simulink model "AcO_Ctrl_Geometric_headless_R2016a"  (R2016a)
settings: Solver=FixedStepDiscrete  StartTime=0.0  StopTime=simulation_duration  FixedStep=Ts  RelTol=1e-3
values from neighbouring files (symbols this model uses):
  M1_BeMo_d = zeros(7,M1_n_mode)    [AcO_Ctrl_headless_cfg.m]    (also in agws_cfg.m = 1e-6*bsxfun(@times,randn(7,M1_n_mode),scale); agws_fastTT_cfg.m = 1e-6*bsxfun(@times,randn(7,M1_n_mode),scale))
  M1_RiBo_d = zeros(7,6)    [AcO_Ctrl_headless_cfg.m]    (also in agws_cfg.m = [M1_Txyz0 M1_Rxyz0]; agws_fastTT_cfg.m = [M1_Txyz0 M1_Rxyz0])
  M2_RiBo_d = zeros(7,6)    [AcO_Ctrl_headless_cfg.m]    (also in agws_cfg.m = [M2_Txyz0 M2_Rxyz0]; agws_fastTT_cfg.m = [M2_Txyz0 M2_Rxyz0])
  Ts = 1/fs    (= 0.002)    [AcO_Ctrl_headless_cfg.m]    (also in agws_fastTT_cfg.m = 0.005)
undefined symbols (not defined in the file or in its folder): Az_C, CG2Hp, CG2Hp_S7, El_C, Fsmm, GIR_C, Hp2CG_f, Hp2CG_f_S7, HPdtf, HpK, KM2, M2_actdyn, M2_CG2Hp, M_LOS, MIMO_C, PTT2act, PTT2act_even, Q, sysd, TT2act, TT2act_even
undefined symbols (not defined in the file): on_axis_src_outputs
libraries: CEO x2
(part 2 of 6)

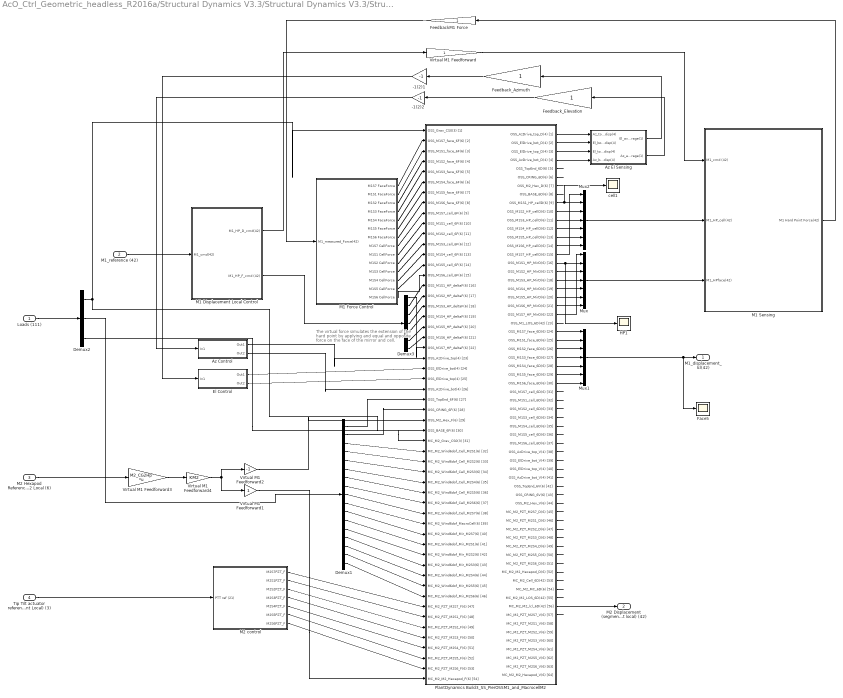
== system AcO_Ctrl_Geometric_headless_R2016a/Structural Dynamics V3.3/Structural Dynamics V3.3/Structural Dynamics Plus CL Az El M1 force ==
  note: The virtual force simulates the extension
      | of the hard point by applying and equal and
      | opposite force on the face of the mirror and cell.
  Loads (111) : Inport
  M1_reference (42) : Inport  Port=2
  M2 Hexapod Reference M2 Local (6) : Inport  Port=3
  Tip Tilt actuator reference (segment Local) (3) : Inport  Port=4
  -1(2)1 : Gain  Gain=-1
  -1(2)2 : Gain  Gain=-1
  Az Control : Subsystem
  Az El Sensing : Subsystem
  Demux1 : Demux  Outputs=6*ones(17,1)
  Demux2 : Demux  Outputs=[3,102,6]
  Demux3 : Demux  Outputs=6*ones(7,1)
  El Control : Subsystem
  Face5 : Scope
  FeedbackM1 Force : Gain
  Feedback_Azimuth : Gain
  Feedback_Elevation : Gain
  HP1 : Scope
  M1 Displacement Local Control : Subsystem
  M1 Force Control : Subsystem
  M1 Sensing : Subsystem
  M2 control : Subsystem
  Mux : Mux  Inputs=6*ones(7,1)
  Mux1 : Mux  Inputs=6*ones(7,1)
  Mux2 : Mux  Inputs=6*ones(7,1)
  PlantDynamics Build3_SS_PierOSSM1_and_MacrocellM2 : Subsystem
  Virtual M1 Feedforward : Gain
  Virtual M1 Feedforward1 : Gain
  Virtual M1 Feedforward2 : Gain  Gain=-1
  Virtual M1 Feedforward3 : Gain  Gain=M2_CG2Hp  Multiplication=Matrix(K*u)
  Virtual M1 Feedforward4 : Gain  Gain=KM2
  cell1 : Scope
  M1_displacement_lcl(42) : Outport
  M2 Displacement (segment local) (42) : Outport  Port=2
  wires:
  Loads (111)/1 -> Demux2/1
  M2 Hexapod Reference M2 Local (6)/1 -> Virtual M1 Feedforward3/1
  PlantDynamics Build3_SS_PierOSSM1_and_MacrocellM2/38(OSS_AzDrive_top_V(4) [38]) -> ?
  Virtual M1 Feedforward4/1 -> Virtual M1 Feedforward1/1, Virtual M1 Feedforward2/1
  Demux1/1 -> PlantDynamics Build3_SS_PierOSSM1_and_MacrocellM2/27(OSS_TopEnd_6F(6) [27])
  M2 control/7(M2S6PZT_F) -> PlantDynamics Build3_SS_PierOSSM1_and_MacrocellM2/53(MC_M2_PZT_M2S6_F(6) [53])
  M2 control/6(M2S5PZT_F) -> PlantDynamics Build3_SS_PierOSSM1_and_MacrocellM2/52(MC_M2_PZT_M2S5_F(6) [52])
  M2 control/5(M2S4PZT_F) -> PlantDynamics Build3_SS_PierOSSM1_and_MacrocellM2/51(MC_M2_PZT_M2S4_F(6) [51])
  M2 control/4(M2S3PZT_F) -> PlantDynamics Build3_SS_PierOSSM1_and_MacrocellM2/50(MC_M2_PZT_M2S3_F(6) [50])
  M2 control/3(M2S2PZT_F) -> PlantDynamics Build3_SS_PierOSSM1_and_MacrocellM2/49(MC_M2_PZT_M2S2_F(6) [49])
  M2 control/2(M2S1PZT_F) -> PlantDynamics Build3_SS_PierOSSM1_and_MacrocellM2/48(MC_M2_PZT_M2S1_F(6) [48])
  M2 control/1(M2S7PZT_F) -> PlantDynamics Build3_SS_PierOSSM1_and_MacrocellM2/47(MC_M2_PZT_M2S7_F(6) [47])
  Tip Tilt actuator reference (segment Local) (3)/1 -> M2 control/1(PTT ref (21))
  Demux3/2 -> PlantDynamics Build3_SS_PierOSSM1_and_MacrocellM2/16(OSS_M1S1_HP_deltaF(6) [16])
  Demux3/7 -> PlantDynamics Build3_SS_PierOSSM1_and_MacrocellM2/21(OSS_M1S6_HP_deltaF(6) [21])
  Demux3/6 -> PlantDynamics Build3_SS_PierOSSM1_and_MacrocellM2/20(OSS_M1S5_HP_deltaF(6) [20])
  Demux3/1 -> PlantDynamics Build3_SS_PierOSSM1_and_MacrocellM2/22(OSS_M1S7_HP_deltaF(6) [22])
  Demux3/4 -> PlantDynamics Build3_SS_PierOSSM1_and_MacrocellM2/18(OSS_M1S3_HP_deltaF(6) [18])
  Demux3/5 -> PlantDynamics Build3_SS_PierOSSM1_and_MacrocellM2/19(OSS_M1S4_HP_deltaF(6) [19])
  Demux3/3 -> PlantDynamics Build3_SS_PierOSSM1_and_MacrocellM2/17(OSS_M1S2_HP_deltaF(6) [17])
  Az El Sensing/2(Az_average(1)) -> Feedback_Elevation/1
  Az El Sensing/1(El_average(1)) -> Feedback_Azimuth/1
  PlantDynamics Build3_SS_PierOSSM1_and_MacrocellM2/3(OSS_ElDrive_top_D(4) [3]) -> Az El Sensing/3(El_top_disp(4))
  PlantDynamics Build3_SS_PierOSSM1_and_MacrocellM2/4(OSS_AzDrive_bot_D(4) [4]) -> Az El Sensing/4(Az_bot_disp(4))
  PlantDynamics Build3_SS_PierOSSM1_and_MacrocellM2/2(OSS_ElDrive_bot_D(4) [2]) -> Az El Sensing/2(El_bottom_disp(4))
  PlantDynamics Build3_SS_PierOSSM1_and_MacrocellM2/1(OSS_AzDrive_top_D(4) [1]) -> Az El Sensing/1(Az_top_disp(4))
  El Control/2(Out2) -> PlantDynamics Build3_SS_PierOSSM1_and_MacrocellM2/25(OSS_ElDrive_top(4) [25])
  El Control/1(Out1) -> PlantDynamics Build3_SS_PierOSSM1_and_MacrocellM2/24(OSS_ElDrive_bot(4) [24])
  -1(2)1/1 -> El Control/1(In1)
  Az Control/2(Out2) -> PlantDynamics Build3_SS_PierOSSM1_and_MacrocellM2/26(OSS_AzDrive_bot(4) [26])
  Az Control/1(Out1) -> PlantDynamics Build3_SS_PierOSSM1_and_MacrocellM2/23(OSS_AzDrive_top(4) [23])
  -1(2)2/1 -> Az Control/1(In1)
  Feedback_Elevation/1 -> -1(2)2/1
  Feedback_Azimuth/1 -> -1(2)1/1
  Demux2/1 -> PlantDynamics Build3_SS_PierOSSM1_and_MacrocellM2/31(MC_M2_Grav_CS0(3) [31]), PlantDynamics Build3_SS_PierOSSM1_and_MacrocellM2/1(OSS_Grav_CS0(3) [1])
  PlantDynamics Build3_SS_PierOSSM1_and_MacrocellM2/21(OSS_M1S6_HP_MirD(6) [21]) -> Mux/7
  PlantDynamics Build3_SS_PierOSSM1_and_MacrocellM2/20(OSS_M1S5_HP_MirD(6) [20]) -> Mux/6
  PlantDynamics Build3_SS_PierOSSM1_and_MacrocellM2/22(OSS_M1S7_HP_MirD(6) [22]) -> Mux/1
  PlantDynamics Build3_SS_PierOSSM1_and_MacrocellM2/18(OSS_M1S3_HP_MirD(6) [18]) -> Mux/4
  PlantDynamics Build3_SS_PierOSSM1_and_MacrocellM2/19(OSS_M1S4_HP_MirD(6) [19]) -> Mux/5
  PlantDynamics Build3_SS_PierOSSM1_and_MacrocellM2/17(OSS_M1S2_HP_MirD(6) [17]) -> Mux/3
  PlantDynamics Build3_SS_PierOSSM1_and_MacrocellM2/16(OSS_M1S1_HP_MirD(6) [16]) -> Mux/2, HP1/1
  PlantDynamics Build3_SS_PierOSSM1_and_MacrocellM2/15(OSS_M1S7_HP_cellD(6) [15]) -> Mux2/1
  PlantDynamics Build3_SS_PierOSSM1_and_MacrocellM2/14(OSS_M1S6_HP_cellD(6) [14]) -> Mux2/7
  PlantDynamics Build3_SS_PierOSSM1_and_MacrocellM2/13(OSS_M1S5_HP_cellD(6) [13]) -> Mux2/6
  PlantDynamics Build3_SS_PierOSSM1_and_MacrocellM2/11(OSS_M1S3_HP_cellD(6) [11]) -> Mux2/4
  PlantDynamics Build3_SS_PierOSSM1_and_MacrocellM2/12(OSS_M1S4_HP_cellD(6) [12]) -> Mux2/5
  PlantDynamics Build3_SS_PierOSSM1_and_MacrocellM2/10(OSS_M1S2_HP_cellD(6) [10]) -> Mux2/3
  PlantDynamics Build3_SS_PierOSSM1_and_MacrocellM2/9(OSS_M1S1_HP_cellD(6) [9]) -> Mux2/2, cell1/1
  PlantDynamics Build3_SS_PierOSSM1_and_MacrocellM2/29(OSS_M1S5_face_6D(6) [29]) -> Mux1/6
  PlantDynamics Build3_SS_PierOSSM1_and_MacrocellM2/30(OSS_M1S6_face_6D(6) [30]) -> Mux1/7
  PlantDynamics Build3_SS_PierOSSM1_and_MacrocellM2/27(OSS_M1S3_face_6D(6) [27]) -> Mux1/4
  PlantDynamics Build3_SS_PierOSSM1_and_MacrocellM2/28(OSS_M1S4_face_6D(6) [28]) -> Mux1/5
  PlantDynamics Build3_SS_PierOSSM1_and_MacrocellM2/25(OSS_M1S1_face_6D(6) [25]) -> Mux1/2
  PlantDynamics Build3_SS_PierOSSM1_and_MacrocellM2/26(OSS_M1S2_face_6D(6) [26]) -> Mux1/3
  PlantDynamics Build3_SS_PierOSSM1_and_MacrocellM2/24(OSS_M1S7_face_6D(6) [24]) -> Mux1/1
  Mux1/1 -> M1_displacement_lcl(42)/1, Face5/1
  Virtual M1 Feedforward/1 -> M1 Sensing/1(M1_cmd (42))
  M1 Displacement Local Control/2(M1_HP_F_cmd (42)) -> Demux3/1
  M1 Displacement Local Control/1(M1_HP_D_cmd(42)) -> Virtual M1 Feedforward/1
  M1_reference (42)/1 -> M1 Displacement Local Control/1(M1_cmd(42))
  M1 Force Control/14(M1S6 CellForce) -> PlantDynamics Build3_SS_PierOSSM1_and_MacrocellM2/15(OSS_M1S6_cell_6F(6) [15])
  M1 Force Control/13(M1S5 CellForce) -> PlantDynamics Build3_SS_PierOSSM1_and_MacrocellM2/14(OSS_M1S5_cell_6F(6) [14])
  M1 Force Control/12(M1S4 CellForce) -> PlantDynamics Build3_SS_PierOSSM1_and_MacrocellM2/13(OSS_M1S4_cell_6F(6) [13])
  M1 Force Control/11(M1S3 CellForce) -> PlantDynamics Build3_SS_PierOSSM1_and_MacrocellM2/12(OSS_M1S3_cell_6F(6) [12])
  M1 Force Control/10(M1S2 CellForce) -> PlantDynamics Build3_SS_PierOSSM1_and_MacrocellM2/11(OSS_M1S2_cell_6F(6) [11])
  M1 Force Control/9(M1S1 CellForce) -> PlantDynamics Build3_SS_PierOSSM1_and_MacrocellM2/10(OSS_M1S1_cell_6F(6) [10])
  M1 Force Control/8(M1S7 CellForce) -> PlantDynamics Build3_SS_PierOSSM1_and_MacrocellM2/9(OSS_M1S7_cell_6F(6) [9])
  M1 Force Control/7(M1S6 FaceForce) -> PlantDynamics Build3_SS_PierOSSM1_and_MacrocellM2/8(OSS_M1S6_face_6F(6) [8])
  M1 Force Control/6(M1S5 FaceForce) -> PlantDynamics Build3_SS_PierOSSM1_and_MacrocellM2/7(OSS_M1S5_face_6F(6) [7])
  M1 Force Control/5(M1S4 FaceForce) -> PlantDynamics Build3_SS_PierOSSM1_and_MacrocellM2/6(OSS_M1S4_face_6F(6) [6])
  M1 Force Control/4(M1S3 FaceForce) -> PlantDynamics Build3_SS_PierOSSM1_and_MacrocellM2/5(OSS_M1S3_face_6F(6) [5])
  M1 Force Control/3(M1S2 FaceForce) -> PlantDynamics Build3_SS_PierOSSM1_and_MacrocellM2/4(OSS_M1S2_face_6F(6) [4])
  M1 Force Control/2(M1S1 FaceForce) -> PlantDynamics Build3_SS_PierOSSM1_and_MacrocellM2/3(OSS_M1S1_face_6F(6) [3])
  M1 Force Control/1(M1S7 FaceForce) -> PlantDynamics Build3_SS_PierOSSM1_and_MacrocellM2/2(OSS_M1S7_face_6F(6) [2])
  FeedbackM1 Force/1 -> M1 Force Control/1(M1_measured_Force(42))
  M1 Sensing/1(M1 Hard Point Force(42)) -> FeedbackM1 Force/1
  Mux2/1 -> M1 Sensing/2(M1_HP_cell(42))
  Mux/1 -> M1 Sensing/3(M1_HPface(42))
  PlantDynamics Build3_SS_PierOSSM1_and_MacrocellM2/7(OSS_M2_Hex_D(6) [7]) -> ?
  Demux1/13 -> PlantDynamics Build3_SS_PierOSSM1_and_MacrocellM2/42(MC_M2_Wind6dof_Mir_M2S2(6) [42])
  Demux1/14 -> PlantDynamics Build3_SS_PierOSSM1_and_MacrocellM2/43(MC_M2_Wind6dof_Mir_M2S3(6) [43])
  Demux2/3 -> PlantDynamics Build3_SS_PierOSSM1_and_MacrocellM2/30(OSS_BASE_6F(6) [30])
  PlantDynamics Build3_SS_PierOSSM1_and_MacrocellM2/35(OSS_M1S4_cell_6D(6) [35]) -> ?
  Demux1/2 -> PlantDynamics Build3_SS_PierOSSM1_and_MacrocellM2/28(OSS_CRING_6F(6) [28])
  PlantDynamics Build3_SS_PierOSSM1_and_MacrocellM2/53(MC_M2_Cell_6D(42) [53]) -> ?
  PlantDynamics Build3_SS_PierOSSM1_and_MacrocellM2/39(OSS_ElDrive_bot_V(4) [39]) -> ?
  PlantDynamics Build3_SS_PierOSSM1_and_MacrocellM2/44(OSS_M2_Hex_V(6) [44]) -> ?
  PlantDynamics Build3_SS_PierOSSM1_and_MacrocellM2/52(MC_M2_M2_Hexapod_D(6) [52]) -> ?
  PlantDynamics Build3_SS_PierOSSM1_and_MacrocellM2/46(MC_M2_PZT_M2S1_D(6) [46]) -> ?
  Demux1/12 -> PlantDynamics Build3_SS_PierOSSM1_and_MacrocellM2/41(MC_M2_Wind6dof_Mir_M2S1(6) [41])
  Demux1/11 -> PlantDynamics Build3_SS_PierOSSM1_and_MacrocellM2/40(MC_M2_Wind6dof_Mir_M2S7(6) [40])
  Demux1/8 -> PlantDynamics Build3_SS_PierOSSM1_and_MacrocellM2/37(MC_M2_Wind6dof_Cell_M2S6(6) [37])
  Demux2/2 -> Demux1/1
  Demux1/7 -> PlantDynamics Build3_SS_PierOSSM1_and_MacrocellM2/36(MC_M2_Wind6dof_Cell_M2S5(6) [36])
  Demux1/4 -> PlantDynamics Build3_SS_PierOSSM1_and_MacrocellM2/33(MC_M2_Wind6dof_Cell_M2S2(6) [33])
  PlantDynamics Build3_SS_PierOSSM1_and_MacrocellM2/33(OSS_M1S2_cell_6D(6) [33]) -> ?
  PlantDynamics Build3_SS_PierOSSM1_and_MacrocellM2/55(MC_M2_M2_LOS_6D(42) [55]) -> ?
  PlantDynamics Build3_SS_PierOSSM1_and_MacrocellM2/45(MC_M2_PZT_M2S7_D(6) [45]) -> ?
  PlantDynamics Build3_SS_PierOSSM1_and_MacrocellM2/47(MC_M2_PZT_M2S2_D(6) [47]) -> ?
  Demux1/17 -> PlantDynamics Build3_SS_PierOSSM1_and_MacrocellM2/46(MC_M2_Wind6dof_Mir_M2S6(6) [46])
  Demux1/10 -> PlantDynamics Build3_SS_PierOSSM1_and_MacrocellM2/39(MC_M2_Wind6dof_MacroCell(6) [39])
  PlantDynamics Build3_SS_PierOSSM1_and_MacrocellM2/36(OSS_M1S5_cell_6D(6) [36]) -> ?
  Demux1/5 -> PlantDynamics Build3_SS_PierOSSM1_and_MacrocellM2/34(MC_M2_Wind6dof_Cell_M2S3(6) [34])
  Demux1/3 -> PlantDynamics Build3_SS_PierOSSM1_and_MacrocellM2/32(MC_M2_Wind6dof_Cell_M2S1(6) [32])
  Demux1/6 -> PlantDynamics Build3_SS_PierOSSM1_and_MacrocellM2/35(MC_M2_Wind6dof_Cell_M2S4(6) [35])
  PlantDynamics Build3_SS_PierOSSM1_and_MacrocellM2/23(OSS_M1_LOS_6D(42) [23]) -> ?
  Virtual M1 Feedforward3/1 -> Virtual M1 Feedforward4/1
  PlantDynamics Build3_SS_PierOSSM1_and_MacrocellM2/57(MC_M2_PZT_M2S7_V(6) [57]) -> ?
  PlantDynamics Build3_SS_PierOSSM1_and_MacrocellM2/49(MC_M2_PZT_M2S4_D(6) [49]) -> ?
  PlantDynamics Build3_SS_PierOSSM1_and_MacrocellM2/8(OSS_BASE_6D(6) [8]) -> ?
  PlantDynamics Build3_SS_PierOSSM1_and_MacrocellM2/34(OSS_M1S3_cell_6D(6) [34]) -> ?
  PlantDynamics Build3_SS_PierOSSM1_and_MacrocellM2/31(OSS_M1S7_cell_6D(6) [31]) -> ?
  PlantDynamics Build3_SS_PierOSSM1_and_MacrocellM2/32(OSS_M1S1_cell_6D(6) [32]) -> ?
  PlantDynamics Build3_SS_PierOSSM1_and_MacrocellM2/48(MC_M2_PZT_M2S3_D(6) [48]) -> ?
  PlantDynamics Build3_SS_PierOSSM1_and_MacrocellM2/6(OSS_CRING_6D(6) [6]) -> ?
  PlantDynamics Build3_SS_PierOSSM1_and_MacrocellM2/54(MC_M2_MC_6D(6) [54]) -> ?
  PlantDynamics Build3_SS_PierOSSM1_and_MacrocellM2/40(OSS_ElDrive_top_V(4) [40]) -> ?
  PlantDynamics Build3_SS_PierOSSM1_and_MacrocellM2/37(OSS_M1S6_cell_6D(6) [37]) -> ?
  Demux1/9 -> PlantDynamics Build3_SS_PierOSSM1_and_MacrocellM2/38(MC_M2_Wind6dof_Cell_M2S7(6) [38])
  PlantDynamics Build3_SS_PierOSSM1_and_MacrocellM2/42(OSS_TopEnd_6V(6) [42]) -> ?
  Virtual M1 Feedforward1/1 -> PlantDynamics Build3_SS_PierOSSM1_and_MacrocellM2/54(MC_M2_M2_Hexapod_F(6) [54])
  PlantDynamics Build3_SS_PierOSSM1_and_MacrocellM2/56(MC_M2_M2_lcl_6D(42) [56]) -> M2 Displacement (segment local) (42)/1
  PlantDynamics Build3_SS_PierOSSM1_and_MacrocellM2/43(OSS_CRING_6V(6) [43]) -> ?
  PlantDynamics Build3_SS_PierOSSM1_and_MacrocellM2/50(MC_M2_PZT_M2S5_D(6) [50]) -> ?
  Virtual M1 Feedforward2/1 -> PlantDynamics Build3_SS_PierOSSM1_and_MacrocellM2/29(OSS_M2_Hex_F(6) [29])
  PlantDynamics Build3_SS_PierOSSM1_and_MacrocellM2/5(OSS_TopEnd_6D(6) [5]) -> ?
  Demux1/15 -> PlantDynamics Build3_SS_PierOSSM1_and_MacrocellM2/44(MC_M2_Wind6dof_Mir_M2S4(6) [44])
  Demux1/16 -> PlantDynamics Build3_SS_PierOSSM1_and_MacrocellM2/45(MC_M2_Wind6dof_Mir_M2S5(6) [45])
  PlantDynamics Build3_SS_PierOSSM1_and_MacrocellM2/41(OSS_AzDrive_bot_V(4) [41]) -> ?
  PlantDynamics Build3_SS_PierOSSM1_and_MacrocellM2/51(MC_M2_PZT_M2S6_D(6) [51]) -> ?

== system AcO_Ctrl_Geometric_headless_R2016a/Structural Dynamics V3.3/Structural Dynamics V3.3a/Loads ==
  " Gravity" : Constant  Value=[0;0;0]
  Base F : Constant  Value=zeros(6,1)
  Mux : Mux  Inputs=[3 102 6]
  Wind : Constant  Value=zeros(17*6,1)
  Out1 : Outport
  wires:
  Mux/1 -> Out1/1
  Base F/1 -> Mux/3
  " Gravity"/1 -> Mux/1
  Wind/1 -> Mux/2

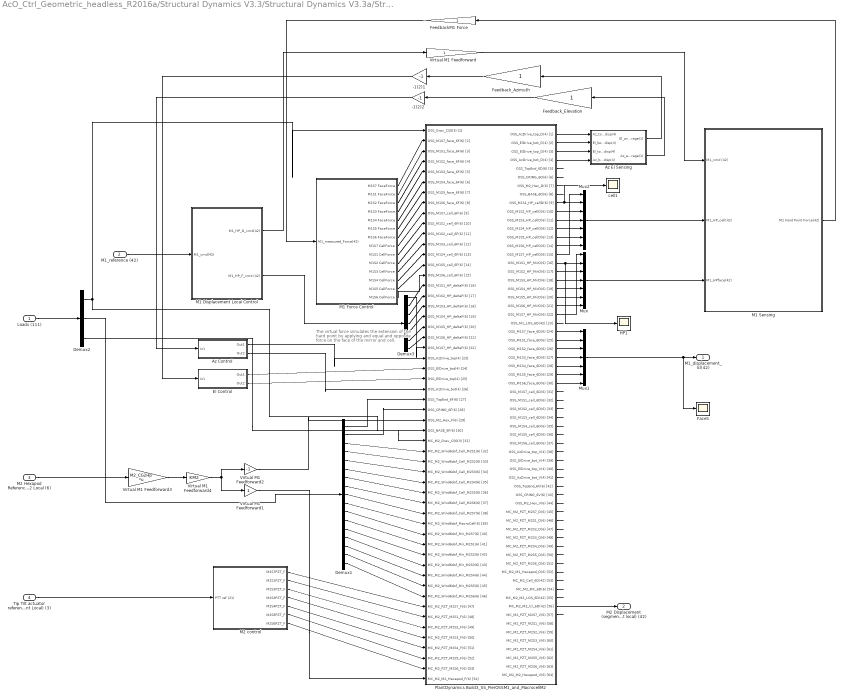
== system AcO_Ctrl_Geometric_headless_R2016a/Structural Dynamics V3.3/Structural Dynamics V3.3a/Structural Dynamics Plus CL Az El M1 force ==
  note: The virtual force simulates the extension
      | of the hard point by applying and equal and
      | opposite force on the face of the mirror and cell.
  Loads (111) : Inport
  M1_reference (42) : Inport  Port=2
  M2 Hexapod Reference M2 Local (6) : Inport  Port=3
  Tip Tilt actuator reference (segment Local) (3) : Inport  Port=4
  -1(2)1 : Gain  Gain=-1
  -1(2)2 : Gain  Gain=-1
  Az Control : Subsystem
  Az El Sensing : Subsystem
  Demux1 : Demux  Outputs=6*ones(17,1)
  Demux2 : Demux  Outputs=[3,102,6]
  Demux3 : Demux  Outputs=6*ones(7,1)
  El Control : Subsystem
  Face5 : Scope
  FeedbackM1 Force : Gain
  Feedback_Azimuth : Gain
  Feedback_Elevation : Gain
  HP1 : Scope
  M1 Displacement Local Control : Subsystem
  M1 Force Control : Subsystem
  M1 Sensing : Subsystem
  M2 control : Subsystem
  Mux : Mux  Inputs=6*ones(7,1)
  Mux1 : Mux  Inputs=6*ones(7,1)
  Mux2 : Mux  Inputs=6*ones(7,1)
  PlantDynamics Build3_SS_PierOSSM1_and_MacrocellM2 : Subsystem
  Virtual M1 Feedforward : Gain
  Virtual M1 Feedforward1 : Gain
  Virtual M1 Feedforward2 : Gain  Gain=-1
  Virtual M1 Feedforward3 : Gain  Gain=M2_CG2Hp  Multiplication=Matrix(K*u)
  Virtual M1 Feedforward4 : Gain  Gain=KM2
  cell1 : Scope
  M1_displacement_lcl(42) : Outport
  M2 Displacement (segment local) (42) : Outport  Port=2
  wires:
  PlantDynamics Build3_SS_PierOSSM1_and_MacrocellM2/51(MC_M2_PZT_M2S6_D(6) [51]) -> ?
  PlantDynamics Build3_SS_PierOSSM1_and_MacrocellM2/41(OSS_AzDrive_bot_V(4) [41]) -> ?
  Demux1/16 -> PlantDynamics Build3_SS_PierOSSM1_and_MacrocellM2/45(MC_M2_Wind6dof_Mir_M2S5(6) [45])
  Demux1/15 -> PlantDynamics Build3_SS_PierOSSM1_and_MacrocellM2/44(MC_M2_Wind6dof_Mir_M2S4(6) [44])
  PlantDynamics Build3_SS_PierOSSM1_and_MacrocellM2/5(OSS_TopEnd_6D(6) [5]) -> ?
  Virtual M1 Feedforward2/1 -> PlantDynamics Build3_SS_PierOSSM1_and_MacrocellM2/29(OSS_M2_Hex_F(6) [29])
  PlantDynamics Build3_SS_PierOSSM1_and_MacrocellM2/50(MC_M2_PZT_M2S5_D(6) [50]) -> ?
  PlantDynamics Build3_SS_PierOSSM1_and_MacrocellM2/43(OSS_CRING_6V(6) [43]) -> ?
  PlantDynamics Build3_SS_PierOSSM1_and_MacrocellM2/56(MC_M2_M2_lcl_6D(42) [56]) -> M2 Displacement (segment local) (42)/1
  Virtual M1 Feedforward1/1 -> PlantDynamics Build3_SS_PierOSSM1_and_MacrocellM2/54(MC_M2_M2_Hexapod_F(6) [54])
  PlantDynamics Build3_SS_PierOSSM1_and_MacrocellM2/42(OSS_TopEnd_6V(6) [42]) -> ?
  Demux1/9 -> PlantDynamics Build3_SS_PierOSSM1_and_MacrocellM2/38(MC_M2_Wind6dof_Cell_M2S7(6) [38])
  PlantDynamics Build3_SS_PierOSSM1_and_MacrocellM2/37(OSS_M1S6_cell_6D(6) [37]) -> ?
  PlantDynamics Build3_SS_PierOSSM1_and_MacrocellM2/40(OSS_ElDrive_top_V(4) [40]) -> ?
  PlantDynamics Build3_SS_PierOSSM1_and_MacrocellM2/54(MC_M2_MC_6D(6) [54]) -> ?
  PlantDynamics Build3_SS_PierOSSM1_and_MacrocellM2/6(OSS_CRING_6D(6) [6]) -> ?
  PlantDynamics Build3_SS_PierOSSM1_and_MacrocellM2/48(MC_M2_PZT_M2S3_D(6) [48]) -> ?
  PlantDynamics Build3_SS_PierOSSM1_and_MacrocellM2/32(OSS_M1S1_cell_6D(6) [32]) -> ?
  PlantDynamics Build3_SS_PierOSSM1_and_MacrocellM2/31(OSS_M1S7_cell_6D(6) [31]) -> ?
  PlantDynamics Build3_SS_PierOSSM1_and_MacrocellM2/34(OSS_M1S3_cell_6D(6) [34]) -> ?
  PlantDynamics Build3_SS_PierOSSM1_and_MacrocellM2/8(OSS_BASE_6D(6) [8]) -> ?
  PlantDynamics Build3_SS_PierOSSM1_and_MacrocellM2/49(MC_M2_PZT_M2S4_D(6) [49]) -> ?
  PlantDynamics Build3_SS_PierOSSM1_and_MacrocellM2/57(MC_M2_PZT_M2S7_V(6) [57]) -> ?
  Virtual M1 Feedforward3/1 -> Virtual M1 Feedforward4/1
  PlantDynamics Build3_SS_PierOSSM1_and_MacrocellM2/23(OSS_M1_LOS_6D(42) [23]) -> ?
  Demux1/6 -> PlantDynamics Build3_SS_PierOSSM1_and_MacrocellM2/35(MC_M2_Wind6dof_Cell_M2S4(6) [35])
  Demux1/3 -> PlantDynamics Build3_SS_PierOSSM1_and_MacrocellM2/32(MC_M2_Wind6dof_Cell_M2S1(6) [32])
  Demux1/5 -> PlantDynamics Build3_SS_PierOSSM1_and_MacrocellM2/34(MC_M2_Wind6dof_Cell_M2S3(6) [34])
  PlantDynamics Build3_SS_PierOSSM1_and_MacrocellM2/36(OSS_M1S5_cell_6D(6) [36]) -> ?
  Demux1/10 -> PlantDynamics Build3_SS_PierOSSM1_and_MacrocellM2/39(MC_M2_Wind6dof_MacroCell(6) [39])
  Demux1/17 -> PlantDynamics Build3_SS_PierOSSM1_and_MacrocellM2/46(MC_M2_Wind6dof_Mir_M2S6(6) [46])
  PlantDynamics Build3_SS_PierOSSM1_and_MacrocellM2/47(MC_M2_PZT_M2S2_D(6) [47]) -> ?
  PlantDynamics Build3_SS_PierOSSM1_and_MacrocellM2/45(MC_M2_PZT_M2S7_D(6) [45]) -> ?
  PlantDynamics Build3_SS_PierOSSM1_and_MacrocellM2/55(MC_M2_M2_LOS_6D(42) [55]) -> ?
  PlantDynamics Build3_SS_PierOSSM1_and_MacrocellM2/33(OSS_M1S2_cell_6D(6) [33]) -> ?
  Demux1/4 -> PlantDynamics Build3_SS_PierOSSM1_and_MacrocellM2/33(MC_M2_Wind6dof_Cell_M2S2(6) [33])
  Demux1/7 -> PlantDynamics Build3_SS_PierOSSM1_and_MacrocellM2/36(MC_M2_Wind6dof_Cell_M2S5(6) [36])
  Demux2/2 -> Demux1/1
  Demux1/8 -> PlantDynamics Build3_SS_PierOSSM1_and_MacrocellM2/37(MC_M2_Wind6dof_Cell_M2S6(6) [37])
  Demux1/11 -> PlantDynamics Build3_SS_PierOSSM1_and_MacrocellM2/40(MC_M2_Wind6dof_Mir_M2S7(6) [40])
  Demux1/12 -> PlantDynamics Build3_SS_PierOSSM1_and_MacrocellM2/41(MC_M2_Wind6dof_Mir_M2S1(6) [41])
  PlantDynamics Build3_SS_PierOSSM1_and_MacrocellM2/46(MC_M2_PZT_M2S1_D(6) [46]) -> ?
  PlantDynamics Build3_SS_PierOSSM1_and_MacrocellM2/52(MC_M2_M2_Hexapod_D(6) [52]) -> ?
  PlantDynamics Build3_SS_PierOSSM1_and_MacrocellM2/44(OSS_M2_Hex_V(6) [44]) -> ?
  PlantDynamics Build3_SS_PierOSSM1_and_MacrocellM2/39(OSS_ElDrive_bot_V(4) [39]) -> ?
  PlantDynamics Build3_SS_PierOSSM1_and_MacrocellM2/53(MC_M2_Cell_6D(42) [53]) -> ?
  Demux1/2 -> PlantDynamics Build3_SS_PierOSSM1_and_MacrocellM2/28(OSS_CRING_6F(6) [28])
  PlantDynamics Build3_SS_PierOSSM1_and_MacrocellM2/35(OSS_M1S4_cell_6D(6) [35]) -> ?
  Demux2/3 -> PlantDynamics Build3_SS_PierOSSM1_and_MacrocellM2/30(OSS_BASE_6F(6) [30])
  Demux1/14 -> PlantDynamics Build3_SS_PierOSSM1_and_MacrocellM2/43(MC_M2_Wind6dof_Mir_M2S3(6) [43])
  Demux1/13 -> PlantDynamics Build3_SS_PierOSSM1_and_MacrocellM2/42(MC_M2_Wind6dof_Mir_M2S2(6) [42])
  PlantDynamics Build3_SS_PierOSSM1_and_MacrocellM2/7(OSS_M2_Hex_D(6) [7]) -> ?
  Mux/1 -> M1 Sensing/3(M1_HPface(42))
  Mux2/1 -> M1 Sensing/2(M1_HP_cell(42))
  M1 Sensing/1(M1 Hard Point Force(42)) -> FeedbackM1 Force/1
  FeedbackM1 Force/1 -> M1 Force Control/1(M1_measured_Force(42))
  M1 Force Control/1(M1S7 FaceForce) -> PlantDynamics Build3_SS_PierOSSM1_and_MacrocellM2/2(OSS_M1S7_face_6F(6) [2])
  M1 Force Control/2(M1S1 FaceForce) -> PlantDynamics Build3_SS_PierOSSM1_and_MacrocellM2/3(OSS_M1S1_face_6F(6) [3])
  M1 Force Control/3(M1S2 FaceForce) -> PlantDynamics Build3_SS_PierOSSM1_and_MacrocellM2/4(OSS_M1S2_face_6F(6) [4])
  M1 Force Control/4(M1S3 FaceForce) -> PlantDynamics Build3_SS_PierOSSM1_and_MacrocellM2/5(OSS_M1S3_face_6F(6) [5])
  M1 Force Control/5(M1S4 FaceForce) -> PlantDynamics Build3_SS_PierOSSM1_and_MacrocellM2/6(OSS_M1S4_face_6F(6) [6])
  M1 Force Control/6(M1S5 FaceForce) -> PlantDynamics Build3_SS_PierOSSM1_and_MacrocellM2/7(OSS_M1S5_face_6F(6) [7])
  M1 Force Control/7(M1S6 FaceForce) -> PlantDynamics Build3_SS_PierOSSM1_and_MacrocellM2/8(OSS_M1S6_face_6F(6) [8])
  M1 Force Control/8(M1S7 CellForce) -> PlantDynamics Build3_SS_PierOSSM1_and_MacrocellM2/9(OSS_M1S7_cell_6F(6) [9])
  M1 Force Control/9(M1S1 CellForce) -> PlantDynamics Build3_SS_PierOSSM1_and_MacrocellM2/10(OSS_M1S1_cell_6F(6) [10])
  M1 Force Control/10(M1S2 CellForce) -> PlantDynamics Build3_SS_PierOSSM1_and_MacrocellM2/11(OSS_M1S2_cell_6F(6) [11])
  M1 Force Control/11(M1S3 CellForce) -> PlantDynamics Build3_SS_PierOSSM1_and_MacrocellM2/12(OSS_M1S3_cell_6F(6) [12])
  M1 Force Control/12(M1S4 CellForce) -> PlantDynamics Build3_SS_PierOSSM1_and_MacrocellM2/13(OSS_M1S4_cell_6F(6) [13])
  M1 Force Control/13(M1S5 CellForce) -> PlantDynamics Build3_SS_PierOSSM1_and_MacrocellM2/14(OSS_M1S5_cell_6F(6) [14])
  M1 Force Control/14(M1S6 CellForce) -> PlantDynamics Build3_SS_PierOSSM1_and_MacrocellM2/15(OSS_M1S6_cell_6F(6) [15])
  M1_reference (42)/1 -> M1 Displacement Local Control/1(M1_cmd(42))
  M1 Displacement Local Control/1(M1_HP_D_cmd(42)) -> Virtual M1 Feedforward/1
  M1 Displacement Local Control/2(M1_HP_F_cmd (42)) -> Demux3/1
  Virtual M1 Feedforward/1 -> M1 Sensing/1(M1_cmd (42))
  Mux1/1 -> Face5/1, M1_displacement_lcl(42)/1
  PlantDynamics Build3_SS_PierOSSM1_and_MacrocellM2/24(OSS_M1S7_face_6D(6) [24]) -> Mux1/1
  PlantDynamics Build3_SS_PierOSSM1_and_MacrocellM2/26(OSS_M1S2_face_6D(6) [26]) -> Mux1/3
  PlantDynamics Build3_SS_PierOSSM1_and_MacrocellM2/25(OSS_M1S1_face_6D(6) [25]) -> Mux1/2
  PlantDynamics Build3_SS_PierOSSM1_and_MacrocellM2/28(OSS_M1S4_face_6D(6) [28]) -> Mux1/5
  PlantDynamics Build3_SS_PierOSSM1_and_MacrocellM2/27(OSS_M1S3_face_6D(6) [27]) -> Mux1/4
  PlantDynamics Build3_SS_PierOSSM1_and_MacrocellM2/30(OSS_M1S6_face_6D(6) [30]) -> Mux1/7
  PlantDynamics Build3_SS_PierOSSM1_and_MacrocellM2/29(OSS_M1S5_face_6D(6) [29]) -> Mux1/6
  PlantDynamics Build3_SS_PierOSSM1_and_MacrocellM2/9(OSS_M1S1_HP_cellD(6) [9]) -> cell1/1, Mux2/2
  PlantDynamics Build3_SS_PierOSSM1_and_MacrocellM2/10(OSS_M1S2_HP_cellD(6) [10]) -> Mux2/3
  PlantDynamics Build3_SS_PierOSSM1_and_MacrocellM2/12(OSS_M1S4_HP_cellD(6) [12]) -> Mux2/5
  PlantDynamics Build3_SS_PierOSSM1_and_MacrocellM2/11(OSS_M1S3_HP_cellD(6) [11]) -> Mux2/4
  PlantDynamics Build3_SS_PierOSSM1_and_MacrocellM2/13(OSS_M1S5_HP_cellD(6) [13]) -> Mux2/6
  PlantDynamics Build3_SS_PierOSSM1_and_MacrocellM2/14(OSS_M1S6_HP_cellD(6) [14]) -> Mux2/7
  PlantDynamics Build3_SS_PierOSSM1_and_MacrocellM2/15(OSS_M1S7_HP_cellD(6) [15]) -> Mux2/1
  PlantDynamics Build3_SS_PierOSSM1_and_MacrocellM2/16(OSS_M1S1_HP_MirD(6) [16]) -> HP1/1, Mux/2
  PlantDynamics Build3_SS_PierOSSM1_and_MacrocellM2/17(OSS_M1S2_HP_MirD(6) [17]) -> Mux/3
  PlantDynamics Build3_SS_PierOSSM1_and_MacrocellM2/19(OSS_M1S4_HP_MirD(6) [19]) -> Mux/5
  PlantDynamics Build3_SS_PierOSSM1_and_MacrocellM2/18(OSS_M1S3_HP_MirD(6) [18]) -> Mux/4
  PlantDynamics Build3_SS_PierOSSM1_and_MacrocellM2/22(OSS_M1S7_HP_MirD(6) [22]) -> Mux/1
  PlantDynamics Build3_SS_PierOSSM1_and_MacrocellM2/20(OSS_M1S5_HP_MirD(6) [20]) -> Mux/6
  PlantDynamics Build3_SS_PierOSSM1_and_MacrocellM2/21(OSS_M1S6_HP_MirD(6) [21]) -> Mux/7
  Demux2/1 -> PlantDynamics Build3_SS_PierOSSM1_and_MacrocellM2/1(OSS_Grav_CS0(3) [1]), PlantDynamics Build3_SS_PierOSSM1_and_MacrocellM2/31(MC_M2_Grav_CS0(3) [31])
  Feedback_Azimuth/1 -> -1(2)1/1
  Feedback_Elevation/1 -> -1(2)2/1
  -1(2)2/1 -> Az Control/1(In1)
  Az Control/1(Out1) -> PlantDynamics Build3_SS_PierOSSM1_and_MacrocellM2/23(OSS_AzDrive_top(4) [23])
  Az Control/2(Out2) -> PlantDynamics Build3_SS_PierOSSM1_and_MacrocellM2/26(OSS_AzDrive_bot(4) [26])
  -1(2)1/1 -> El Control/1(In1)
  El Control/1(Out1) -> PlantDynamics Build3_SS_PierOSSM1_and_MacrocellM2/24(OSS_ElDrive_bot(4) [24])
  El Control/2(Out2) -> PlantDynamics Build3_SS_PierOSSM1_and_MacrocellM2/25(OSS_ElDrive_top(4) [25])
  PlantDynamics Build3_SS_PierOSSM1_and_MacrocellM2/1(OSS_AzDrive_top_D(4) [1]) -> Az El Sensing/1(Az_top_disp(4))
  PlantDynamics Build3_SS_PierOSSM1_and_MacrocellM2/2(OSS_ElDrive_bot_D(4) [2]) -> Az El Sensing/2(El_bottom_disp(4))
  PlantDynamics Build3_SS_PierOSSM1_and_MacrocellM2/4(OSS_AzDrive_bot_D(4) [4]) -> Az El Sensing/4(Az_bot_disp(4))
  PlantDynamics Build3_SS_PierOSSM1_and_MacrocellM2/3(OSS_ElDrive_top_D(4) [3]) -> Az El Sensing/3(El_top_disp(4))
  Az El Sensing/1(El_average(1)) -> Feedback_Azimuth/1
  Az El Sensing/2(Az_average(1)) -> Feedback_Elevation/1
  Demux3/3 -> PlantDynamics Build3_SS_PierOSSM1_and_MacrocellM2/17(OSS_M1S2_HP_deltaF(6) [17])
  Demux3/5 -> PlantDynamics Build3_SS_PierOSSM1_and_MacrocellM2/19(OSS_M1S4_HP_deltaF(6) [19])
  Demux3/4 -> PlantDynamics Build3_SS_PierOSSM1_and_MacrocellM2/18(OSS_M1S3_HP_deltaF(6) [18])
  Demux3/1 -> PlantDynamics Build3_SS_PierOSSM1_and_MacrocellM2/22(OSS_M1S7_HP_deltaF(6) [22])
  Demux3/6 -> PlantDynamics Build3_SS_PierOSSM1_and_MacrocellM2/20(OSS_M1S5_HP_deltaF(6) [20])
  Demux3/7 -> PlantDynamics Build3_SS_PierOSSM1_and_MacrocellM2/21(OSS_M1S6_HP_deltaF(6) [21])
  Demux3/2 -> PlantDynamics Build3_SS_PierOSSM1_and_MacrocellM2/16(OSS_M1S1_HP_deltaF(6) [16])
  Tip Tilt actuator reference (segment Local) (3)/1 -> M2 control/1(PTT ref (21))
  M2 control/1(M2S7PZT_F) -> PlantDynamics Build3_SS_PierOSSM1_and_MacrocellM2/47(MC_M2_PZT_M2S7_F(6) [47])
  M2 control/2(M2S1PZT_F) -> PlantDynamics Build3_SS_PierOSSM1_and_MacrocellM2/48(MC_M2_PZT_M2S1_F(6) [48])
  M2 control/3(M2S2PZT_F) -> PlantDynamics Build3_SS_PierOSSM1_and_MacrocellM2/49(MC_M2_PZT_M2S2_F(6) [49])
  M2 control/4(M2S3PZT_F) -> PlantDynamics Build3_SS_PierOSSM1_and_MacrocellM2/50(MC_M2_PZT_M2S3_F(6) [50])
  M2 control/5(M2S4PZT_F) -> PlantDynamics Build3_SS_PierOSSM1_and_MacrocellM2/51(MC_M2_PZT_M2S4_F(6) [51])
  M2 control/6(M2S5PZT_F) -> PlantDynamics Build3_SS_PierOSSM1_and_MacrocellM2/52(MC_M2_PZT_M2S5_F(6) [52])
  M2 control/7(M2S6PZT_F) -> PlantDynamics Build3_SS_PierOSSM1_and_MacrocellM2/53(MC_M2_PZT_M2S6_F(6) [53])
  Demux1/1 -> PlantDynamics Build3_SS_PierOSSM1_and_MacrocellM2/27(OSS_TopEnd_6F(6) [27])
  Virtual M1 Feedforward4/1 -> Virtual M1 Feedforward2/1, Virtual M1 Feedforward1/1
  PlantDynamics Build3_SS_PierOSSM1_and_MacrocellM2/38(OSS_AzDrive_top_V(4) [38]) -> ?
  M2 Hexapod Reference M2 Local (6)/1 -> Virtual M1 Feedforward3/1
  Loads (111)/1 -> Demux2/1

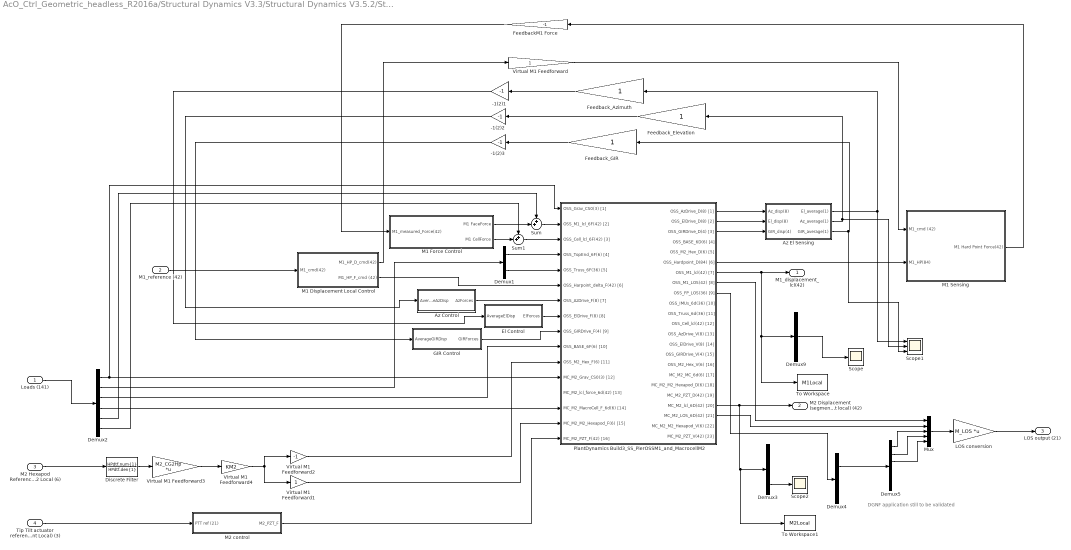
== system AcO_Ctrl_Geometric_headless_R2016a/Structural Dynamics V3.3/Structural Dynamics V3.5.2/Structural Dynamics Plus CL Az El M1 force ==
  note: DGNF application still to be validated
  Loads (141) : Inport
  M1_reference (42) : Inport  Port=2
  M2 Hexapod Reference M2 Local (6) : Inport  Port=3
  Tip Tilt actuator reference (segment Local) (3) : Inport  Port=4
  -1(2)1 : Gain  Gain=-1
  -1(2)2 : Gain  Gain=-1
  -1(2)3 : Gain  Gain=-1
  Az Control : Subsystem
  Az El Sensing : Subsystem
  Demux1 : Demux  Outputs=[6,36]
  Demux2 : Demux  Outputs=[3,42,6,6,42,42]
  Demux3 : Demux  Outputs=[6,30,6]
  Demux4 : Demux  Outputs=6*ones(6,1)
  Demux5 : Demux  Outputs=6
  Demux9 : Demux  Outputs=[6,6,30]
  Discrete Filter : DiscreteFilter  Numerator=HPdtf.num{1}  Denominator=HPdtf.den{1}
  El Control : Subsystem
  FeedbackM1 Force : Gain  Gain=-1
  Feedback_Azimuth : Gain
  Feedback_Elevation : Gain
  Feedback_GIR : Gain
  GIR Control : Subsystem
  LOS conversion : Gain  Gain=M_LOS  Multiplication=Matrix(K*u)
  M1 Displacement Local Control : Subsystem
  M1 Force Control : Subsystem
  M1 Sensing : Subsystem
  M2 control : Subsystem
  Mux : Mux  Inputs=[42 42 1 1 1]
  PlantDynamics Build3_SS_PierOSSM1_and_MacrocellM2 : Subsystem
  Scope : Scope
  Scope1 : Scope  NumInputPorts=3
  Scope2 : Scope
  Sum : Sum  Inputs=++|
  Sum1 : Sum  Inputs=++|
  To Workspace : ToWorkspace  VariableName=M1Local  SaveFormat=Timeseries  SampleTime=-1
  To Workspace1 : ToWorkspace  VariableName=M2Local  SaveFormat=Timeseries  SampleTime=-1
  Virtual M1 Feedforward : Gain
  Virtual M1 Feedforward1 : Gain
  Virtual M1 Feedforward2 : Gain  Gain=-1
  Virtual M1 Feedforward3 : Gain  Gain=M2_CG2Hp  Multiplication=Matrix(K*u)
  Virtual M1 Feedforward4 : Gain  Gain=KM2
  M1_displacement_lcl(42) : Outport
  M2 Displacement (segment local) (42) : Outport  Port=2
  LOS output (21) : Outport  Port=3
  wires:
  Virtual M1 Feedforward3/1 -> Virtual M1 Feedforward4/1
  Demux2/2 -> Demux1/1
  PlantDynamics Build3_SS_PierOSSM1_and_MacrocellM2/6(OSS_Hardpoint_D(84) [6]) -> M1 Sensing/2(M1_HP(84))
  M1 Sensing/1(M1 Hard Point Force(42)) -> FeedbackM1 Force/1
  FeedbackM1 Force/1 -> M1 Force Control/1(M1_measured_Force(42))
  M1_reference (42)/1 -> M1 Displacement Local Control/1(M1_cmd(42))
  M1 Displacement Local Control/1(M1_HP_D_cmd(42)) -> Virtual M1 Feedforward/1
  M1 Displacement Local Control/2(M1_HP_F_cmd (42)) -> PlantDynamics Build3_SS_PierOSSM1_and_MacrocellM2/6(OSS_Harpoint_delta_F(42) [6])
  Virtual M1 Feedforward/1 -> M1 Sensing/1(M1_cmd (42))
  Demux2/1 -> PlantDynamics Build3_SS_PierOSSM1_and_MacrocellM2/1(OSS_Grav_CS0(3) [1]), PlantDynamics Build3_SS_PierOSSM1_and_MacrocellM2/12(MC_M2_Grav_CS0(3) [12])
  Feedback_Azimuth/1 -> -1(2)1/1
  Feedback_Elevation/1 -> -1(2)2/1
  -1(2)2/1 -> Az Control/1(AverageAzDisp)
  -1(2)1/1 -> El Control/1(AverageElDisp)
  Az El Sensing/1(El_average(1)) -> Scope1/1, Feedback_Azimuth/1
  Az El Sensing/2(Az_average(1)) -> Scope1/2, Feedback_Elevation/1
  Tip Tilt actuator reference (segment Local) (3)/1 -> M2 control/1(PTT ref (21))
  Virtual M1 Feedforward4/1 -> Virtual M1 Feedforward2/1, Virtual M1 Feedforward1/1
  M2 Hexapod Reference M2 Local (6)/1 -> Discrete Filter/1
  Loads (141)/1 -> Demux2/1
  M1 Force Control/1(M1 FaceForce) -> Sum/2
  Demux2/4 -> PlantDynamics Build3_SS_PierOSSM1_and_MacrocellM2/14(MC_M2_MacroCell_F_6d(6) [14])
  Demux1/2 -> PlantDynamics Build3_SS_PierOSSM1_and_MacrocellM2/5(OSS_Truss_6F(36) [5])
  Demux1/1 -> PlantDynamics Build3_SS_PierOSSM1_and_MacrocellM2/4(OSS_TopEnd_6F(6) [4])
  Az Control/1(AzForces) -> PlantDynamics Build3_SS_PierOSSM1_and_MacrocellM2/7(OSS_AzDrive_F(8) [7])
  El Control/1(ElForces) -> PlantDynamics Build3_SS_PierOSSM1_and_MacrocellM2/8(OSS_ElDrive_F(8) [8])
  Demux2/3 -> PlantDynamics Build3_SS_PierOSSM1_and_MacrocellM2/10(OSS_BASE_6F(6) [10])
  Virtual M1 Feedforward2/1 -> PlantDynamics Build3_SS_PierOSSM1_and_MacrocellM2/11(OSS_M2_Hex_F(6) [11])
  Virtual M1 Feedforward1/1 -> PlantDynamics Build3_SS_PierOSSM1_and_MacrocellM2/15(MC_M2_M2_Hexapod_F(6) [15])
  M2 control/1(M2_PZT_F) -> PlantDynamics Build3_SS_PierOSSM1_and_MacrocellM2/16(MC_M2_PZT_F(42) [16])
  PlantDynamics Build3_SS_PierOSSM1_and_MacrocellM2/1(OSS_AzDrive_D(8) [1]) -> Az El Sensing/1(Az_disp(8))
  PlantDynamics Build3_SS_PierOSSM1_and_MacrocellM2/2(OSS_ElDrive_D(8) [2]) -> Az El Sensing/2(El_disp(8))
  PlantDynamics Build3_SS_PierOSSM1_and_MacrocellM2/3(OSS_GIRDrive_D(4) [3]) -> Az El Sensing/3(GIR_disp(4))
  PlantDynamics Build3_SS_PierOSSM1_and_MacrocellM2/7(OSS_M1_lcl(42) [7]) -> To Workspace/1, Demux9/1, M1_displacement_lcl(42)/1
  GIR Control/1(GIRForces) -> PlantDynamics Build3_SS_PierOSSM1_and_MacrocellM2/9(OSS_GIRDrive_F(4) [9])
  Feedback_GIR/1 -> -1(2)3/1
  Az El Sensing/3(GIR_average(1)) -> Scope1/3, Feedback_GIR/1
  -1(2)3/1 -> GIR Control/1(AverageGIRDisp)
  Demux9/2 -> Scope/1
  PlantDynamics Build3_SS_PierOSSM1_and_MacrocellM2/20(MC_M2_lcl_6D(42) [20]) -> To Workspace1/1, Demux3/1, M2 Displacement (segment local) (42)/1
  Demux3/3 -> Scope2/1
  PlantDynamics Build3_SS_PierOSSM1_and_MacrocellM2/21(MC_M2_LOS_6D(42) [21]) -> Mux/2
  M1 Force Control/2(M1 CellForce) -> Sum1/2
  Sum1/1 -> PlantDynamics Build3_SS_PierOSSM1_and_MacrocellM2/3(OSS_Cell_lcl_6F(42) [3])
  Sum/1 -> PlantDynamics Build3_SS_PierOSSM1_and_MacrocellM2/2(OSS_M1_lcl_6F(42) [2])
  Demux2/5 -> Sum/1
  Demux2/6 -> Sum1/1
  Mux/1 -> LOS conversion/1
  PlantDynamics Build3_SS_PierOSSM1_and_MacrocellM2/8(OSS_M1_LOS(42) [8]) -> Mux/1
  PlantDynamics Build3_SS_PierOSSM1_and_MacrocellM2/9(OSS_FP_LOS(36) [9]) -> Demux4/1
  Demux4/2 -> Demux5/1
  Demux5/1 -> Mux/3
  Demux5/2 -> Mux/4
  Demux5/3 -> Mux/5
  LOS conversion/1 -> LOS output (21)/1
  Discrete Filter/1 -> Virtual M1 Feedforward3/1

== system AcO_Ctrl_Geometric_headless_R2016a/Structural Dynamics V3.3/Structural Dynamics V3.5.2/Windloads ==
  note: Red are the IM random loads
  " Gravity" : Constant  Value=[0;0;0]
  Base Force : Constant  Value=zeros(6,1)
  M1 : Constant  Value=zeros(42,1)
  M1Cell(42) : FromWorkspace  VariableName=M1CellLoads  SampleTime=0
  M1Mirror(42) : FromWorkspace  VariableName=M1MirrorLoads  SampleTime=0
  M2 : Constant  Value=zeros(6,1)
  M2(6) : FromWorkspace  VariableName=M2Loads  SampleTime=0
  Manual Switch{,2..6} (6 alike) : ManualSwitch  CurrentSetting=0
  Manual Switch1 : ManualSwitch
  Mux : Mux  Inputs=[3 6 36 6 6 42 42]
  TE(6) : Constant  Value=zeros(6,1)
  Truss : Constant  Value=zeros(36,1)
  Truss(36) : FromWorkspace  VariableName=TrussLoads  SampleTime=0
  LoadInputs : Outport
  wires:
  Manual Switch/1 -> Mux/1
  Mux/1 -> LoadInputs/1
  " Gravity"/1 -> Manual Switch/2, Manual Switch/1
  TE(6)/1 -> Manual Switch1/2, Manual Switch1/1
  Manual Switch1/1 -> Mux/2
  Manual Switch2/1 -> Mux/3
  Manual Switch3/1 -> Mux/4
  Manual Switch4/1 -> Mux/5
  Truss/1 -> Manual Switch2/2
  Truss(36)/1 -> Manual Switch2/1
  Base Force/1 -> Manual Switch3/1, Manual Switch3/2
  M2/1 -> Manual Switch4/2
  M2(6)/1 -> Manual Switch4/1
  Manual Switch5/1 -> Mux/6
  Manual Switch6/1 -> Mux/7
  M1/1 -> Manual Switch6/2, Manual Switch5/2
  M1Mirror(42)/1 -> Manual Switch5/1
  M1Cell(42)/1 -> Manual Switch6/1

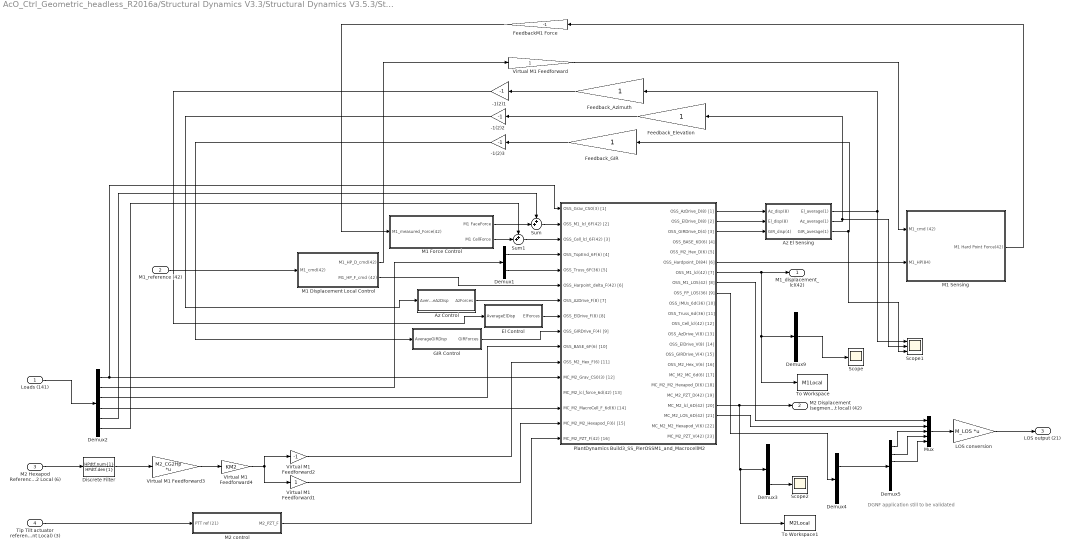
== system AcO_Ctrl_Geometric_headless_R2016a/Structural Dynamics V3.3/Structural Dynamics V3.5.3/Structural Dynamics Plus CL Az El M1 force ==
  note: DGNF application still to be validated
  Loads (141) : Inport
  M1_reference (42) : Inport  Port=2
  M2 Hexapod Reference M2 Local (6) : Inport  Port=3
  Tip Tilt actuator reference (segment Local) (3) : Inport  Port=4
  -1(2)1 : Gain  Gain=-1
  -1(2)2 : Gain  Gain=-1
  -1(2)3 : Gain  Gain=-1
  Az Control : Subsystem
  Az El Sensing : Subsystem
  Demux1 : Demux  Outputs=[6,36]
  Demux2 : Demux  Outputs=[3,42,6,6,42,42]
  Demux3 : Demux  Outputs=[6,30,6]
  Demux4 : Demux  Outputs=6*ones(6,1)
  Demux5 : Demux  Outputs=6
  Demux9 : Demux  Outputs=[6,6,30]
  Discrete Filter : DiscreteFilter  Numerator=HPdtf.num{1}  Denominator=HPdtf.den{1}
  El Control : Subsystem
  FeedbackM1 Force : Gain  Gain=-1
  Feedback_Azimuth : Gain
  Feedback_Elevation : Gain
  Feedback_GIR : Gain
  GIR Control : Subsystem
  LOS conversion : Gain  Gain=M_LOS  Multiplication=Matrix(K*u)
  M1 Displacement Local Control : Subsystem
  M1 Force Control : Subsystem
  M1 Sensing : Subsystem
  M2 control : Subsystem
  Mux : Mux  Inputs=[42 42 1 1 1]
  PlantDynamics Build3_SS_PierOSSM1_and_MacrocellM2 : Subsystem
  Scope : Scope
  Scope1 : Scope  NumInputPorts=3
  Scope2 : Scope
  Sum : Sum  Inputs=++|
  Sum1 : Sum  Inputs=++|
  To Workspace : ToWorkspace  VariableName=M1Local  SaveFormat=Timeseries  SampleTime=-1
  To Workspace1 : ToWorkspace  VariableName=M2Local  SaveFormat=Timeseries  SampleTime=-1
  Virtual M1 Feedforward : Gain
  Virtual M1 Feedforward1 : Gain
  Virtual M1 Feedforward2 : Gain  Gain=-1
  Virtual M1 Feedforward3 : Gain  Gain=M2_CG2Hp  Multiplication=Matrix(K*u)
  Virtual M1 Feedforward4 : Gain  Gain=KM2
  M1_displacement_lcl(42) : Outport
  M2 Displacement (segment local) (42) : Outport  Port=2
  LOS output (21) : Outport  Port=3
  wires:
  Virtual M1 Feedforward3/1 -> Virtual M1 Feedforward4/1
  Demux2/2 -> Demux1/1
  PlantDynamics Build3_SS_PierOSSM1_and_MacrocellM2/6(OSS_Hardpoint_D(84) [6]) -> M1 Sensing/2(M1_HP(84))
  M1 Sensing/1(M1 Hard Point Force(42)) -> FeedbackM1 Force/1
  FeedbackM1 Force/1 -> M1 Force Control/1(M1_measured_Force(42))
  M1_reference (42)/1 -> M1 Displacement Local Control/1(M1_cmd(42))
  M1 Displacement Local Control/1(M1_HP_D_cmd(42)) -> Virtual M1 Feedforward/1
  M1 Displacement Local Control/2(M1_HP_F_cmd (42)) -> PlantDynamics Build3_SS_PierOSSM1_and_MacrocellM2/6(OSS_Harpoint_delta_F(42) [6])
  Virtual M1 Feedforward/1 -> M1 Sensing/1(M1_cmd (42))
  Demux2/1 -> PlantDynamics Build3_SS_PierOSSM1_and_MacrocellM2/1(OSS_Grav_CS0(3) [1]), PlantDynamics Build3_SS_PierOSSM1_and_MacrocellM2/12(MC_M2_Grav_CS0(3) [12])
  Feedback_Azimuth/1 -> -1(2)1/1
  Feedback_Elevation/1 -> -1(2)2/1
  -1(2)2/1 -> Az Control/1(AverageAzDisp)
  -1(2)1/1 -> El Control/1(AverageElDisp)
  Az El Sensing/1(El_average(1)) -> Scope1/1, Feedback_Azimuth/1
  Az El Sensing/2(Az_average(1)) -> Scope1/2, Feedback_Elevation/1
  Tip Tilt actuator reference (segment Local) (3)/1 -> M2 control/1(PTT ref (21))
  Virtual M1 Feedforward4/1 -> Virtual M1 Feedforward2/1, Virtual M1 Feedforward1/1
  M2 Hexapod Reference M2 Local (6)/1 -> Discrete Filter/1
  Loads (141)/1 -> Demux2/1
  M1 Force Control/1(M1 FaceForce) -> Sum/2
  Demux2/4 -> PlantDynamics Build3_SS_PierOSSM1_and_MacrocellM2/14(MC_M2_MacroCell_F_6d(6) [14])
  Demux1/2 -> PlantDynamics Build3_SS_PierOSSM1_and_MacrocellM2/5(OSS_Truss_6F(36) [5])
  Demux1/1 -> PlantDynamics Build3_SS_PierOSSM1_and_MacrocellM2/4(OSS_TopEnd_6F(6) [4])
  Az Control/1(AzForces) -> PlantDynamics Build3_SS_PierOSSM1_and_MacrocellM2/7(OSS_AzDrive_F(8) [7])
  El Control/1(ElForces) -> PlantDynamics Build3_SS_PierOSSM1_and_MacrocellM2/8(OSS_ElDrive_F(8) [8])
  Demux2/3 -> PlantDynamics Build3_SS_PierOSSM1_and_MacrocellM2/10(OSS_BASE_6F(6) [10])
  Virtual M1 Feedforward2/1 -> PlantDynamics Build3_SS_PierOSSM1_and_MacrocellM2/11(OSS_M2_Hex_F(6) [11])
  Virtual M1 Feedforward1/1 -> PlantDynamics Build3_SS_PierOSSM1_and_MacrocellM2/15(MC_M2_M2_Hexapod_F(6) [15])
  M2 control/1(M2_PZT_F) -> PlantDynamics Build3_SS_PierOSSM1_and_MacrocellM2/16(MC_M2_PZT_F(42) [16])
  PlantDynamics Build3_SS_PierOSSM1_and_MacrocellM2/1(OSS_AzDrive_D(8) [1]) -> Az El Sensing/1(Az_disp(8))
  PlantDynamics Build3_SS_PierOSSM1_and_MacrocellM2/2(OSS_ElDrive_D(8) [2]) -> Az El Sensing/2(El_disp(8))
  PlantDynamics Build3_SS_PierOSSM1_and_MacrocellM2/3(OSS_GIRDrive_D(4) [3]) -> Az El Sensing/3(GIR_disp(4))
  PlantDynamics Build3_SS_PierOSSM1_and_MacrocellM2/7(OSS_M1_lcl(42) [7]) -> To Workspace/1, Demux9/1, M1_displacement_lcl(42)/1
  GIR Control/1(GIRForces) -> PlantDynamics Build3_SS_PierOSSM1_and_MacrocellM2/9(OSS_GIRDrive_F(4) [9])
  Feedback_GIR/1 -> -1(2)3/1
  Az El Sensing/3(GIR_average(1)) -> Scope1/3, Feedback_GIR/1
  -1(2)3/1 -> GIR Control/1(AverageGIRDisp)
  Demux9/2 -> Scope/1
  PlantDynamics Build3_SS_PierOSSM1_and_MacrocellM2/20(MC_M2_lcl_6D(42) [20]) -> To Workspace1/1, Demux3/1, M2 Displacement (segment local) (42)/1
  Demux3/3 -> Scope2/1
  PlantDynamics Build3_SS_PierOSSM1_and_MacrocellM2/21(MC_M2_LOS_6D(42) [21]) -> Mux/2
  M1 Force Control/2(M1 CellForce) -> Sum1/2
  Sum1/1 -> PlantDynamics Build3_SS_PierOSSM1_and_MacrocellM2/3(OSS_Cell_lcl_6F(42) [3])
  Sum/1 -> PlantDynamics Build3_SS_PierOSSM1_and_MacrocellM2/2(OSS_M1_lcl_6F(42) [2])
  Demux2/5 -> Sum/1
  Demux2/6 -> Sum1/1
  Mux/1 -> LOS conversion/1
  PlantDynamics Build3_SS_PierOSSM1_and_MacrocellM2/8(OSS_M1_LOS(42) [8]) -> Mux/1
  PlantDynamics Build3_SS_PierOSSM1_and_MacrocellM2/9(OSS_FP_LOS(36) [9]) -> Demux4/1
  Demux4/2 -> Demux5/1
  Demux5/1 -> Mux/3
  Demux5/2 -> Mux/4
  Demux5/3 -> Mux/5
  LOS conversion/1 -> LOS output (21)/1
  Discrete Filter/1 -> Virtual M1 Feedforward3/1

== system AcO_Ctrl_Geometric_headless_R2016a/Structural Dynamics V3.3/Structural Dynamics V3.5.3/Windloads ==
  note: Red are the IM random loads
  " Gravity" : Constant  Value=[0;0;0]
  Base Force : Constant  Value=zeros(6,1)
  M1 : Constant  Value=zeros(42,1)
  M1Cell(42) : FromWorkspace  VariableName=M1CellLoads  SampleTime=0
  M1Mirror(42) : FromWorkspace  VariableName=M1MirrorLoads  SampleTime=0
  M2 : Constant  Value=zeros(6,1)
  M2(6) : FromWorkspace  VariableName=M2Loads  SampleTime=0
  Manual Switch : ManualSwitch  CurrentSetting=0
  Manual Switch{1..2,4..6} (5 alike) : ManualSwitch
  Manual Switch3 : ManualSwitch  CurrentSetting=0
  Mux : Mux  Inputs=[3 6 36 6 6 42 42]
  TE(6) : Constant  Value=zeros(6,1)
  Truss : Constant  Value=zeros(36,1)
  Truss(36) : FromWorkspace  VariableName=TrussLoads  SampleTime=0
  LoadInputs : Outport
  wires:
  Manual Switch/1 -> Mux/1
  Mux/1 -> LoadInputs/1
  " Gravity"/1 -> Manual Switch/2, Manual Switch/1
  TE(6)/1 -> Manual Switch1/2, Manual Switch1/1
  Manual Switch1/1 -> Mux/2
  Manual Switch2/1 -> Mux/3
  Manual Switch3/1 -> Mux/4
  Manual Switch4/1 -> Mux/5
  Truss/1 -> Manual Switch2/2
  Truss(36)/1 -> Manual Switch2/1
  Base Force/1 -> Manual Switch3/1, Manual Switch3/2
  M2/1 -> Manual Switch4/2
  M2(6)/1 -> Manual Switch4/1
  Manual Switch5/1 -> Mux/6
  Manual Switch6/1 -> Mux/7
  M1/1 -> Manual Switch6/2, Manual Switch5/2
  M1Mirror(42)/1 -> Manual Switch5/1
  M1Cell(42)/1 -> Manual Switch6/1

== system AcO_Ctrl_Geometric_headless_R2016a/Structural Dynamics V3.3/Structural Dynamics V3.1/M1 Force Control/ControlM1S1 ==
  In1 : Inport
  -1(2)3 : Gain  Gain=-1
  Actuator Model : DiscreteStateSpace  A=Q.A  B=Q.B  C=Q.C  D=Q.D  SampleTime=1/Fsmm
  MIMO Controller : Subsystem
  Out1 : Outport
  Out2 : Outport  Port=2
  wires:
  MIMO Controller/1(Out1) -> Actuator Model/1
  -1(2)3/1 -> Out2/1
  Actuator Model/1 -> -1(2)3/1, Out1/1
  In1/1 -> MIMO Controller/1(In1)

== system AcO_Ctrl_Geometric_headless_R2016a/Structural Dynamics V3.3/Structural Dynamics V3.1/M1 Force Control/ControlM1S2 ==
  In1 : Inport
  -1(2)3 : Gain  Gain=-1
  Actuator Model : DiscreteStateSpace  A=Q.A  B=Q.B  C=Q.C  D=Q.D  SampleTime=1/Fsmm
  MIMO Controller : Subsystem
  Out1 : Outport
  Out2 : Outport  Port=2
  wires:
  In1/1 -> MIMO Controller/1(In1)
  Actuator Model/1 -> Out1/1, -1(2)3/1
  -1(2)3/1 -> Out2/1
  MIMO Controller/1(Out1) -> Actuator Model/1

== system AcO_Ctrl_Geometric_headless_R2016a/Structural Dynamics V3.3/Structural Dynamics V3.1/M1 Force Control/ControlM1S3 ==
  In1 : Inport
  -1(2)3 : Gain  Gain=-1
  Actuator Model : DiscreteStateSpace  A=Q.A  B=Q.B  C=Q.C  D=Q.D  SampleTime=1/Fsmm
  MIMO Controller : Subsystem
  Out1 : Outport
  Out2 : Outport  Port=2
  wires:
  MIMO Controller/1(Out1) -> Actuator Model/1
  -1(2)3/1 -> Out2/1
  Actuator Model/1 -> -1(2)3/1, Out1/1
  In1/1 -> MIMO Controller/1(In1)

== system AcO_Ctrl_Geometric_headless_R2016a/Structural Dynamics V3.3/Structural Dynamics V3.1/M1 Force Control/ControlM1S4 ==
  In1 : Inport
  -1(2)3 : Gain  Gain=-1
  Actuator Model : DiscreteStateSpace  A=Q.A  B=Q.B  C=Q.C  D=Q.D  SampleTime=1/Fsmm
  MIMO Controller : Subsystem
  Out1 : Outport
  Out2 : Outport  Port=2
  wires:
  In1/1 -> MIMO Controller/1(In1)
  Actuator Model/1 -> Out1/1, -1(2)3/1
  -1(2)3/1 -> Out2/1
  MIMO Controller/1(Out1) -> Actuator Model/1

== system AcO_Ctrl_Geometric_headless_R2016a/Structural Dynamics V3.3/Structural Dynamics V3.1/M1 Force Control/ControlM1S5 ==
  In1 : Inport
  -1(2)3 : Gain  Gain=-1
  Actuator Model : DiscreteStateSpace  A=Q.A  B=Q.B  C=Q.C  D=Q.D  SampleTime=1/Fsmm
  MIMO Controller : Subsystem
  Out1 : Outport
  Out2 : Outport  Port=2
  wires:
  MIMO Controller/1(Out1) -> Actuator Model/1
  -1(2)3/1 -> Out2/1
  Actuator Model/1 -> -1(2)3/1, Out1/1
  In1/1 -> MIMO Controller/1(In1)

== system AcO_Ctrl_Geometric_headless_R2016a/Structural Dynamics V3.3/Structural Dynamics V3.1/M1 Force Control/ControlM1S6 ==
  In1 : Inport
  -1(2)3 : Gain  Gain=-1
  Actuator Model : DiscreteStateSpace  A=Q.A  B=Q.B  C=Q.C  D=Q.D  SampleTime=1/Fsmm
  MIMO Controller : Subsystem
  Out1 : Outport
  Out2 : Outport  Port=2
  wires:
  In1/1 -> MIMO Controller/1(In1)
  Actuator Model/1 -> Out1/1, -1(2)3/1
  -1(2)3/1 -> Out2/1
  MIMO Controller/1(Out1) -> Actuator Model/1

== system AcO_Ctrl_Geometric_headless_R2016a/Structural Dynamics V3.3/Structural Dynamics V3.1/M1 Force Control/ControlM1S7 ==
  In1 : Inport
  -1(2)3 : Gain  Gain=-1
  Actuator Model : DiscreteStateSpace  A=Q.A  B=Q.B  C=Q.C  D=Q.D  SampleTime=1/Fsmm
  MIMO Controller : Subsystem
  Out1 : Outport
  Out2 : Outport  Port=2
  wires:
  MIMO Controller/1(Out1) -> Actuator Model/1
  -1(2)3/1 -> Out2/1
  Actuator Model/1 -> -1(2)3/1, Out1/1
  In1/1 -> MIMO Controller/1(In1)

== system AcO_Ctrl_Geometric_headless_R2016a/Structural Dynamics V3.3/Structural Dynamics V3.1/M1 Sensing/senseM1S1 ==
  6dof_D_cmd : Inport
  6dof_D_face : Inport  Port=2
  6dof_D_cell : Inport  Port=3
  KHp : Gain  Gain=-HpK  Multiplication=Matrix(K*u)
  M1 6dof(relative) : Scope
  Sum9 : Sum  Inputs=--+|
  HardPointForce : Outport
  wires:
  Sum9/1 -> KHp/1, M1 6dof(relative)/1
  6dof_D_cell/1 -> Sum9/1
  6dof_D_cmd/1 -> Sum9/2
  6dof_D_face/1 -> Sum9/3
  KHp/1 -> HardPointForce/1

== system AcO_Ctrl_Geometric_headless_R2016a/Structural Dynamics V3.3/Structural Dynamics V3.1/M1 Sensing/senseM1S2 ==
  6dof_D_cmd : Inport
  6dof_D_face : Inport  Port=2
  6dof_D_cell : Inport  Port=3
  KHp : Gain  Gain=-HpK  Multiplication=Matrix(K*u)
  M1 6dof(relative) : Scope
  Sum9 : Sum  Inputs=--+|
  HardPointForce : Outport
  wires:
  KHp/1 -> HardPointForce/1
  6dof_D_face/1 -> Sum9/3
  6dof_D_cmd/1 -> Sum9/2
  6dof_D_cell/1 -> Sum9/1
  Sum9/1 -> M1 6dof(relative)/1, KHp/1

== system AcO_Ctrl_Geometric_headless_R2016a/Structural Dynamics V3.3/Structural Dynamics V3.1/M1 Sensing/senseM1S3 ==
  6dof_D_cmd : Inport
  6dof_D_face : Inport  Port=2
  6dof_D_cell : Inport  Port=3
  KHp : Gain  Gain=-HpK  Multiplication=Matrix(K*u)
  M1 6dof(relative) : Scope
  Sum9 : Sum  Inputs=--+|
  HardPointForce : Outport
  wires:
  Sum9/1 -> KHp/1, M1 6dof(relative)/1
  6dof_D_cell/1 -> Sum9/1
  6dof_D_cmd/1 -> Sum9/2
  6dof_D_face/1 -> Sum9/3
  KHp/1 -> HardPointForce/1

== system AcO_Ctrl_Geometric_headless_R2016a/Structural Dynamics V3.3/Structural Dynamics V3.1/M1 Sensing/senseM1S4 ==
  6dof_D_cmd : Inport
  6dof_D_face : Inport  Port=2
  6dof_D_cell : Inport  Port=3
  KHp : Gain  Gain=-HpK  Multiplication=Matrix(K*u)
  M1 6dof(relative) : Scope
  Sum9 : Sum  Inputs=--+|
  HardPointForce : Outport
  wires:
  KHp/1 -> HardPointForce/1
  6dof_D_face/1 -> Sum9/3
  6dof_D_cmd/1 -> Sum9/2
  6dof_D_cell/1 -> Sum9/1
  Sum9/1 -> M1 6dof(relative)/1, KHp/1

== system AcO_Ctrl_Geometric_headless_R2016a/Structural Dynamics V3.3/Structural Dynamics V3.1/M1 Sensing/senseM1S5 ==
  6dof_D_cmd : Inport
  6dof_D_face : Inport  Port=2
  6dof_D_cell : Inport  Port=3
  KHp : Gain  Gain=-HpK  Multiplication=Matrix(K*u)
  M1 6dof(relative) : Scope
  Sum9 : Sum  Inputs=--+|
  HardPointForce : Outport
  wires:
  Sum9/1 -> KHp/1, M1 6dof(relative)/1
  6dof_D_cell/1 -> Sum9/1
  6dof_D_cmd/1 -> Sum9/2
  6dof_D_face/1 -> Sum9/3
  KHp/1 -> HardPointForce/1

== system AcO_Ctrl_Geometric_headless_R2016a/Structural Dynamics V3.3/Structural Dynamics V3.1/M1 Sensing/senseM1S6 ==
  6dof_D_cmd : Inport
  6dof_D_face : Inport  Port=2
  6dof_D_cell : Inport  Port=3
  KHp : Gain  Gain=-HpK  Multiplication=Matrix(K*u)
  M1 6dof(relative) : Scope
  Sum9 : Sum  Inputs=--+|
  HardPointForce : Outport
  wires:
  KHp/1 -> HardPointForce/1
  6dof_D_face/1 -> Sum9/3
  6dof_D_cmd/1 -> Sum9/2
  6dof_D_cell/1 -> Sum9/1
  Sum9/1 -> M1 6dof(relative)/1, KHp/1

== system AcO_Ctrl_Geometric_headless_R2016a/Structural Dynamics V3.3/Structural Dynamics V3.1/M1 Sensing/senseM1S7 ==
  6dof_D_cmd : Inport
  6dof_D_face : Inport  Port=2
  6dof_D_cell : Inport  Port=3
  KHp : Gain  Gain=-HpK  Multiplication=Matrix(K*u)
  M1 6dof(relative) : Scope
  Sum9 : Sum  Inputs=--+|
  HardPointForce : Outport
  wires:
  Sum9/1 -> KHp/1, M1 6dof(relative)/1
  6dof_D_cell/1 -> Sum9/1
  6dof_D_cmd/1 -> Sum9/2
  6dof_D_face/1 -> Sum9/3
  KHp/1 -> HardPointForce/1
